simulink model "aquaMasterModel"  (R2023b)
settings: Solver=VariableStepAuto  StartTime=0.0  StopTime=Tfinal  MaxStep=0.25  RelTol=1e-3
settings Model: Creator=kristopherriordan  LastModifiedBy=annahylbert

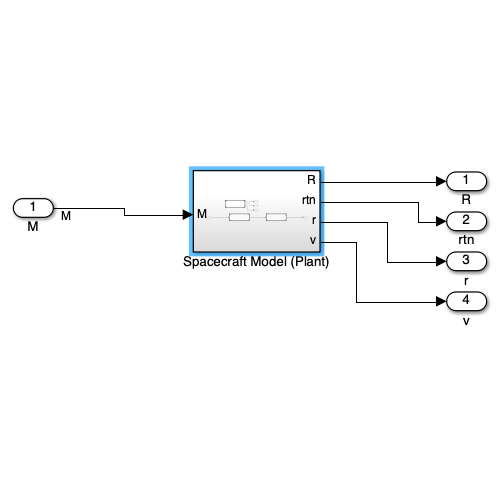
[thumbnail: Simulink's stored preview of the top-level diagram]
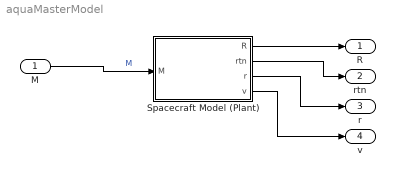
== system aquaMasterModel ==
  M : Inport
  Spacecraft Model (Plant) : Subsystem
  R : Outport
  rtn : Outport  Port=2
  r : Outport  Port=3
  v : Outport  Port=4
  wires:
  M/1 -> Spacecraft Model (Plant)/1(M)  "M"
  Spacecraft Model (Plant)/1(R) -> R/1
  Spacecraft Model (Plant)/2(rtn) -> rtn/1
  Spacecraft Model (Plant)/3(r) -> r/1
  Spacecraft Model (Plant)/4(v) -> v/1

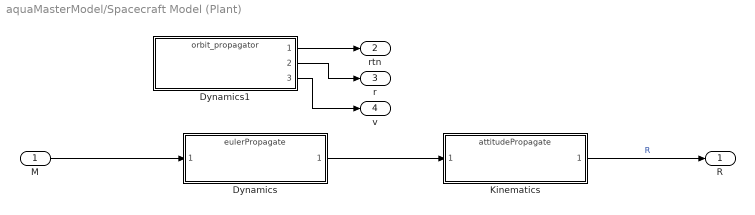
== system aquaMasterModel/Spacecraft Model (Plant) ==
  M : Inport
  Dynamics : ModelReference  ModelNameDialog=eulerPropagate.slx  SimulationMode=Normal  ModelReferenceVersion=1.30
  Dynamics1 : ModelReference  ModelNameDialog=orbit_propagator.slx  SimulationMode=Normal  ModelReferenceVersion=1.12
  Kinematics : ModelReference  ModelNameDialog=attitudePropagate.slx  SimulationMode=Normal  ModelReferenceVersion=1.19
  R : Outport
  rtn : Outport  Port=2
  r : Outport  Port=3
  v : Outport  Port=4
  wires:
  Kinematics/1 -> R/1  "R"
  Dynamics/1 -> Kinematics/1
  M/1 -> Dynamics/1
  Dynamics1/1 -> rtn/1
  Dynamics1/2 -> r/1
  Dynamics1/3 -> v/1
